simulink model "Hardware_Model_Position_Control"  (R2023a)
settings: Solver=FixedStepAuto  StartTime=0.0  StopTime=10.0  RelTol=1e-3  EnableMultiTasking=on
undefined symbols (not defined in the file): Ad, Bd, Cd, ki, Kp, L, Ts
settings Model: ExtModeTrigDuration=10  Creator=Marco  LastModifiedBy=Marco
settings OptimizationCC: EnhancedBackFolding=on  PassReuseOutputArgsAs=Individual arguments  ZeroExternalMemoryAtStartup=off  ZeroInternalMemoryAtStartup=off  MaxStackSize=64  OptimizeBlockOrder=speed  DifferentSizesBufferReuse=on  OptimizationCustomize=off  EfficientTunableParamExpr=on
settings DebuggingCC: ParameterTunabilityLossMsg=error
settings HardwareCC: ProdBitPerPointer=32  ProdBitPerSizeT=32  ProdBitPerPtrDiffT=32  ProdLargestAtomicInteger=Long  ProdLargestAtomicFloat=Double  ProdWordSize=32  ProdLongLongMode=on  ProdHWDeviceType=ARM Compatible->ARM Cortex
settings SFSimCC: MATLABDynamicMemAlloc=off
settings RTWCC: Description=Embedded Coder  SystemTargetFile=ert.tlc  HardwareBoard=STM32 Nucleo F401RE  TemplateMakefile=ert_default_tmf  Toolchain=GNU Tools for ARM Embedded Processors  PortableWordSizes=on
settings CodeAppCC: ForceParamTrailComments=on  IgnoreCustomStorageClasses=off  OperatorAnnotations=on  SimulinkDataObjDesc=on  SFDataObjDesc=on  InsertBlockDesc=on
settings ERTTargetCC: ExtModeTransport=3  ExtModeStaticAlloc=on  ExtModeStaticAllocSize=2000  ExtModeMexFile=ext_xcp  ExtModeIntrfLevel=Level2 - Open

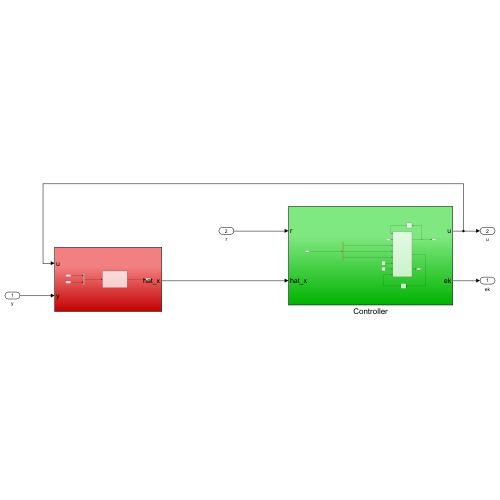
[thumbnail: Simulink's stored preview of the top-level diagram]
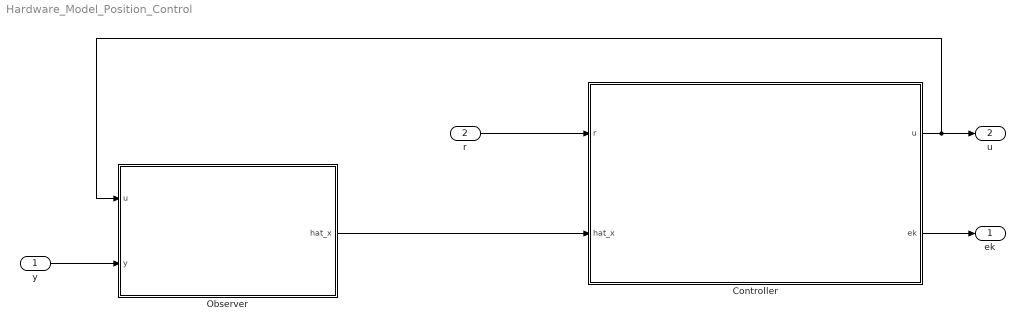
== system Hardware_Model_Position_Control ==
  y : Inport
  r : Inport  Port=2
  Controller : Subsystem
  Observer : Subsystem
  ek : Outport
  u : Outport  Port=2
  wires:
  Observer/1(hat_x) -> Controller/2(hat_x)
  y/1 -> Observer/2(y)
  r/1 -> Controller/1(r)
  Controller/2(ek) -> ek/1
  Controller/1(u) -> Observer/1(u), u/1

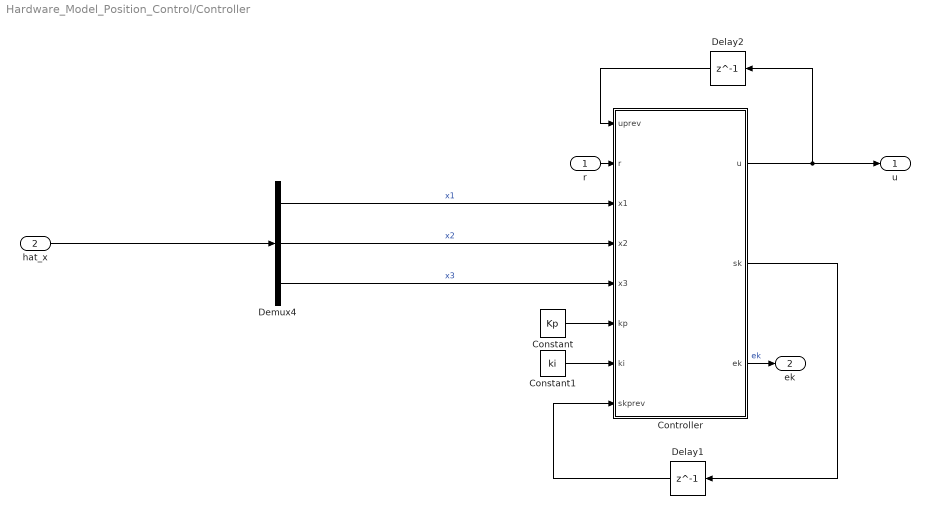
== system Hardware_Model_Position_Control/Controller ==
  r : Inport
  hat_x : Inport  Port=2
  Constant : Constant  Value=Kp  SampleTime=Ts
  Constant1 : Constant  Value=ki  SampleTime=Ts
  Controller : MATLAB Function  TreatAsAtomicUnit=on
  Delay1 : Delay  DelayLength=1  InitialCondition=0  SampleTime=Ts
  Delay2 : Delay  DelayLength=1  InitialCondition=0  SampleTime=Ts
  Demux4 : Demux  Outputs=3
  u : Outport
  ek : Outport  Port=2
  wires:
  Constant/1 -> Controller/6(kp)
  Delay1/1 -> Controller/8(skprev)
  Demux4/2 -> Controller/4(x2)  "x2"
  Delay2/1 -> Controller/1(uprev)
  Demux4/3 -> Controller/5(x3)  "x3"
  r/1 -> Controller/2(r)
  Demux4/1 -> Controller/3(x1)  "x1"
  Controller/2(sk) -> Delay1/1
  Constant1/1 -> Controller/7(ki)
  Controller/1(u) -> u/1, Delay2/1
  Controller/3(ek) -> ek/1  "ek"
  hat_x/1 -> Demux4/1

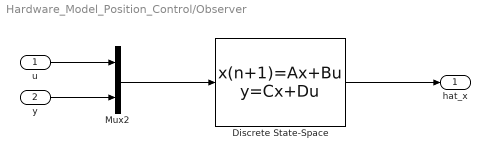
== system Hardware_Model_Position_Control/Observer ==
  u : Inport
  y : Inport  Port=2
  Discrete State-Space : DiscreteStateSpace  A=Ad-L*Cd  B=[Bd L]  C=eye(3)  D=[ 0 0; 0 0; 0 0]  SampleTime=Ts
  Mux2 : Mux  Inputs=2
  hat_x : Outport
  wires:
  Mux2/1 -> Discrete State-Space/1
  u/1 -> Mux2/1
  Discrete State-Space/1 -> hat_x/1
  y/1 -> Mux2/2

== matlab function Hardware_Model_Position_Control/Controller/Controller ==
  data: uprev input; r input; x1 input; u output; x2 input; x3 input; kp input; ki input; skprev input; sk output; ek output
function [u,sk, ek] = fcn(uprev, r, x1, x2, x3, kp, ki, skprev)

ek = r-x1
umax = 12

stopsumm = ((uprev > umax & ek > 0) | (uprev < -umax & ek < 0));

if ~(stopsumm)
   sk = skprev + ek
   u = -kp(1)*(x1) - kp(2)*x2 - kp(3)*x3 + ki*sk;
else
   u = -kp(1)*(x1) - kp(2)*x2 - kp(3)*x3 + ki*skprev;
   sk = skprev
end
